simulink model "asenkronmodeli"  (Simulink 7.7)
settings: Solver=ode45  StartTime=0.0  StopTime=10.0  RelTol=1e-3
values from neighbouring files (symbols this model uses):
  J = 0.0226    [asenkronparametreler.m]
  p = 4    [asenkronparametreler.m]
  Rr = .39    (= 0.39)    [asenkronparametreler.m]
  Rs = .19    (= 0.19)    [asenkronparametreler.m]
  wb = 2*pi*fb    (= 628.318530718)    [asenkronparametreler.m]
  Xlr = wb*Llr    (= 0.376991118431)    [asenkronparametreler.m]
  Xls = wb*Lls    (= 0.131946891451)    [asenkronparametreler.m]
  Xmstar = 1/(1/Xls+1/Xm+1/Xlr)    (= 0.0940797800005)    [asenkronparametreler.m]
settings Model: Creator=Murat  LastModifiedBy=Murat
settings DataIOCC: SignalLoggingSaveFormat=Dataset
settings OptimizationCC: ExpressionDepthLimit=128
settings DebuggingCC: UnderspecifiedInitializationDetection=Simplified  MergeDetectMultiDrivingBlocksExec=error  FcnCallInpInsideContextMsg=Enable All  StateNameClashWarn=none
settings CodeAppCC: CustomSymbolStrType=$N$R$M_T
settings GRTTargetCC: TargetFunctionLibrary=C89/C90 (ANSI)

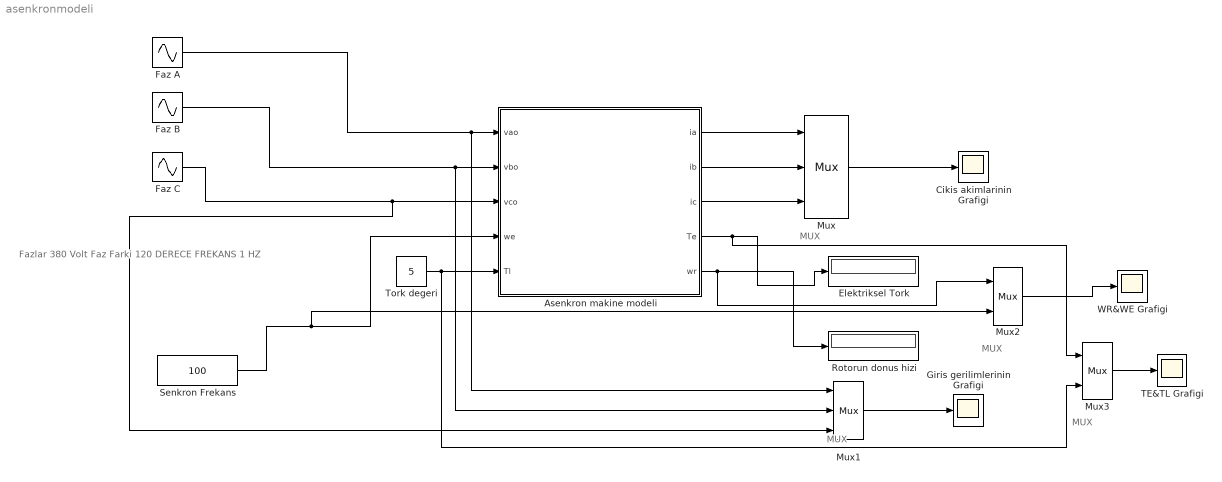
== system asenkronmodeli ==
  note: MUX
  note: MUX
  note: MUX
  note: MUX
  note: Fazlar 380 Volt
      | Faz Farki 120 DERECE
      | FREKANS 1 HZ
  Asenkron makine modeli : Subsystem
  Cikis akimlarinin Grafigi : Scope
      settings: SaveName=ScopeData3
  Elektriksel Tork : Display
  Faz A : Sin  Amplitude=380  SampleTime=0
  Faz B : Sin  Amplitude=380  Phase=(2*pi)/3  SampleTime=0
  Faz C : Sin  Amplitude=380  Phase=(4*pi)/3  SampleTime=0
  Giris gerilimlerinin Grafigi : Scope
      settings: SaveName=ScopeData4
  Mux : Mux  Inputs=3
  Mux1 : Mux  Inputs=3
  Mux2 : Mux  Inputs=2
  Mux3 : Mux  Inputs=2
  Rotorun donus hizi : Display
  Senkron Frekans : Constant  Value=100
  TE&TL Grafigi : Scope
      settings: SaveName=ScopeData5
  Tork degeri : Constant  Value=5
  WR&WE Grafigi : Scope
      settings: SaveName=ScopeData6
  wires:
  Asenkron makine modeli/1(ia) -> Mux/1
  Asenkron makine modeli/2(ib) -> Mux/2
  Asenkron makine modeli/3(ic) -> Mux/3
  Mux/1 -> Cikis akimlarinin Grafigi/1
  Asenkron makine modeli/5(wr) -> Mux2/1, Rotorun donus hizi/1
  Asenkron makine modeli/4(Te) -> Mux3/1, Elektriksel Tork/1
  Mux1/1 -> Giris gerilimlerinin Grafigi/1
  Tork degeri/1 -> Mux3/2, Asenkron makine modeli/5(Tl)
  Senkron Frekans/1 -> Mux2/2, Asenkron makine modeli/4(we)
  Faz A/1 -> Mux1/1, Asenkron makine modeli/1(vao)
  Faz B/1 -> Mux1/2, Asenkron makine modeli/2(vbo)
  Faz C/1 -> Mux1/3, Asenkron makine modeli/3(vco)
  Mux2/1 -> WR&WE Grafigi/1
  Mux3/1 -> TE&TL Grafigi/1

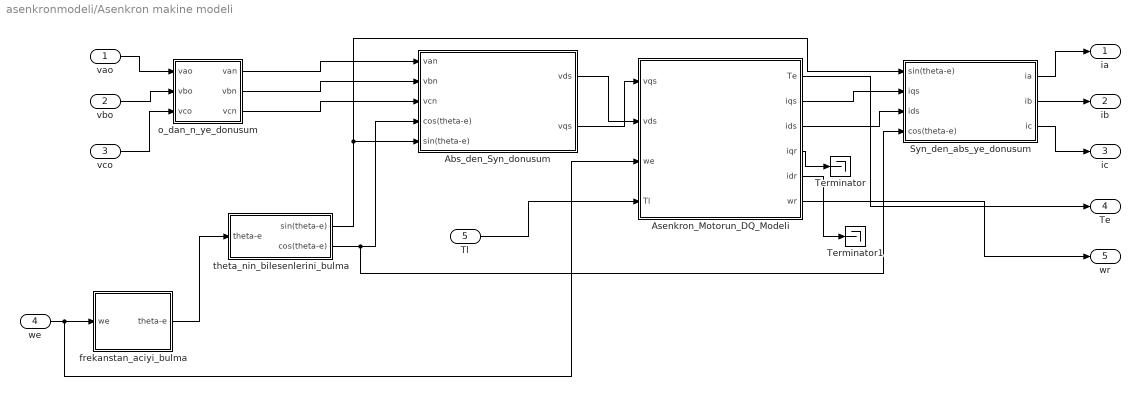
== system asenkronmodeli/Asenkron makine modeli ==
  vao : Inport
  vbo : Inport  Port=2
  vco : Inport  Port=3
  we : Inport  Port=4
  Tl : Inport  Port=5
  Abs_den_Syn_donusum : Subsystem
  Asenkron_Motorun_DQ_Modeli : Subsystem
  Syn_den_abs_ye_donusum : Subsystem
  Terminator : Terminator
  Terminator1 : Terminator
  frekanstan_aciyi_bulma : Subsystem
  o_dan_n_ye_donusum : Subsystem
  theta_nin_bilesenlerini_bulma : Subsystem
  ia : Outport
  ib : Outport  Port=2
  ic : Outport  Port=3
  Te : Outport  Port=4
  wr : Outport  Port=5
  wires:
  vbo/1 -> o_dan_n_ye_donusum/2(vbo)
  vao/1 -> o_dan_n_ye_donusum/1(vao)
  vco/1 -> o_dan_n_ye_donusum/3(vco)
  we/1 -> Asenkron_Motorun_DQ_Modeli/3(we), frekanstan_aciyi_bulma/1(we)
  frekanstan_aciyi_bulma/1(theta-e) -> theta_nin_bilesenlerini_bulma/1(theta-e)
  Asenkron_Motorun_DQ_Modeli/3(ids) -> Syn_den_abs_ye_donusum/3(ids)
  Syn_den_abs_ye_donusum/1(ia) -> ia/1
  Asenkron_Motorun_DQ_Modeli/4(iqr) -> Terminator/1
  Asenkron_Motorun_DQ_Modeli/5(idr) -> Terminator1/1
  Syn_den_abs_ye_donusum/3(ic) -> ic/1
  o_dan_n_ye_donusum/3(vcn) -> Abs_den_Syn_donusum/3(vcn)
  Asenkron_Motorun_DQ_Modeli/2(iqs) -> Syn_den_abs_ye_donusum/2(iqs)
  Abs_den_Syn_donusum/1(vds) -> Asenkron_Motorun_DQ_Modeli/2(vds)
  Abs_den_Syn_donusum/2(vqs) -> Asenkron_Motorun_DQ_Modeli/1(vqs)
  Syn_den_abs_ye_donusum/2(ib) -> ib/1
  Tl/1 -> Asenkron_Motorun_DQ_Modeli/4(Tl)
  o_dan_n_ye_donusum/2(vbn) -> Abs_den_Syn_donusum/2(vbn)
  o_dan_n_ye_donusum/1(van) -> Abs_den_Syn_donusum/1(van)
  Asenkron_Motorun_DQ_Modeli/1(Te) -> Te/1
  Asenkron_Motorun_DQ_Modeli/6(wr) -> wr/1
  theta_nin_bilesenlerini_bulma/2("cos(theta-e)   ") -> Syn_den_abs_ye_donusum/4("cos(theta-e) "), Abs_den_Syn_donusum/4("cos(theta-e) ")
  theta_nin_bilesenlerini_bulma/1("sin(theta-e)  ") -> Syn_den_abs_ye_donusum/1("sin(theta-e)  "), Abs_den_Syn_donusum/5(sin(theta-e))

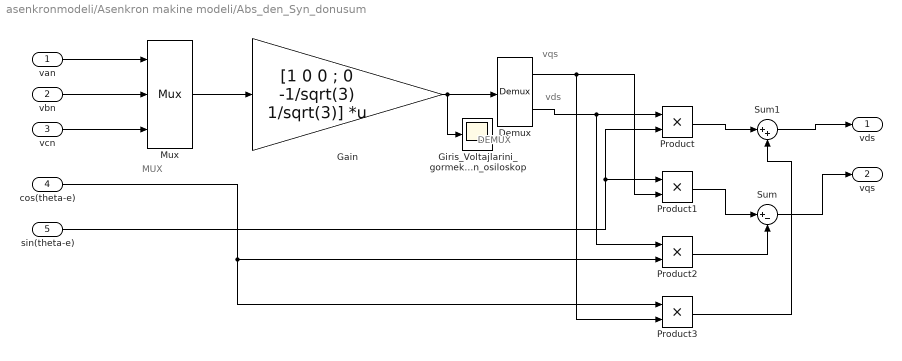
== system asenkronmodeli/Asenkron makine modeli/Abs_den_Syn_donusum ==
  note: vds
  note: vqs
  note: DEMUX
  note: MUX
  van : Inport
  vbn : Inport  Port=2
  vcn : Inport  Port=3
  "cos(theta-e) " : Inport  Port=4
  sin(theta-e) : Inport  Port=5
  Demux : Demux  Outputs=2
  Gain : Gain  Gain="[1 0 0 ; 0 -1/sqrt(3)  1/sqrt(3)]"  Multiplication=Matrix(K*u)  SaturateOnIntegerOverflow=on
  Giris_Voltajlarini_gormek_icin_osiloskop : Scope
  Mux : Mux  Inputs=3
  Product{,1..3} (4 alike) : Product
  Sum : Sum  Inputs=|+-
  Sum1 : Sum  Inputs=|++
  vds : Outport
  vqs : Outport  Port=2
  wires:
  van/1 -> Mux/1
  vbn/1 -> Mux/2
  vcn/1 -> Mux/3
  Mux/1 -> Gain/1
  Gain/1 -> Demux/1, Giris_Voltajlarini_gormek_icin_osiloskop/1
  sin(theta-e)/1 -> Product/2, Product1/1
  "cos(theta-e) "/1 -> Product3/1, Product2/2
  Demux/1 -> Product3/2, Product1/2
  Demux/2 -> Product2/1, Product/1
  Product2/1 -> Sum/2
  Product1/1 -> Sum/1
  Product/1 -> Sum1/1
  Product3/1 -> Sum1/2
  Sum1/1 -> vds/1
  Sum/1 -> vqs/1

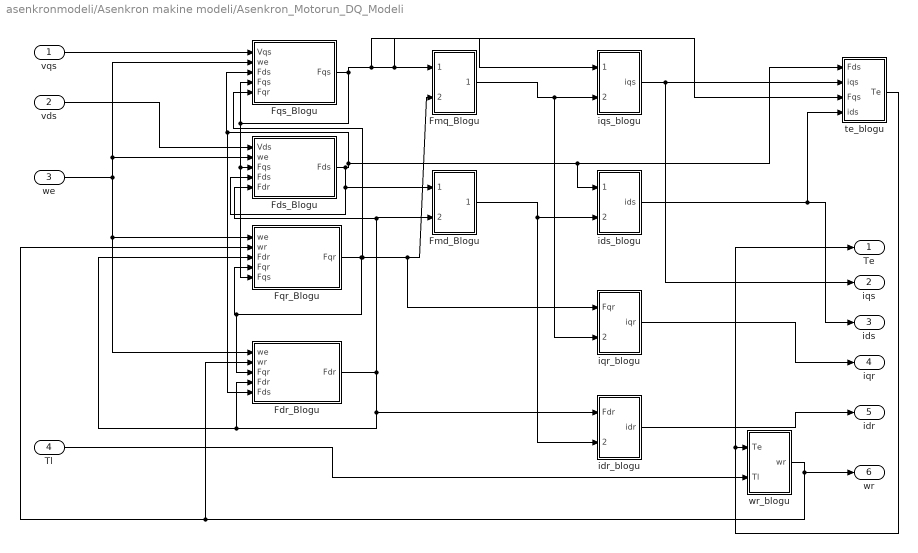
== system asenkronmodeli/Asenkron makine modeli/Asenkron_Motorun_DQ_Modeli ==
  vqs : Inport
  vds : Inport  Port=2
  we : Inport  Port=3
  Tl : Inport  Port=4
  Fdr_Blogu : Subsystem
  Fds_Blogu : Subsystem
  Fmd_Blogu : Subsystem
  Fmq_Blogu : Subsystem
  Fqr_Blogu : Subsystem
  Fqs_Blogu : Subsystem
  idr_blogu : Subsystem
  ids_blogu : Subsystem
  iqr_blogu : Subsystem
  iqs_blogu : Subsystem
  te_blogu : Subsystem
  wr_blogu : Subsystem
  Te : Outport
  iqs : Outport  Port=2
  ids : Outport  Port=3
  iqr : Outport  Port=4
  idr : Outport  Port=5
  wr : Outport  Port=6
  wires:
  vqs/1 -> Fqs_Blogu/1(Vqs)
  vds/1 -> Fds_Blogu/1("Vds ")
  we/1 -> Fds_Blogu/2(we), Fqs_Blogu/2(we), Fdr_Blogu/1("we "), Fqr_Blogu/1("we ")
  Tl/1 -> wr_blogu/2(Tl)
  Fqs_Blogu/1("Fqs   ") -> Fqr_Blogu/5(Fqs), Fds_Blogu/3("Fqs  "), Fqs_Blogu/4(Fqs), te_blogu/3("Fqs  "), iqs_blogu/1(Fqs), Fmq_Blogu/1("Fqs  ")
  Fds_Blogu/1("Fds   ") -> Fmd_Blogu/1("Fds  "), Fds_Blogu/4(Fds), te_blogu/1("Fds   "), ids_blogu/1("Fds  "), Fdr_Blogu/5(Fds), Fqs_Blogu/3(Fds)
  Fqr_Blogu/1("Fqr  ") -> iqr_blogu/1("Fqr  "), Fmq_Blogu/2("Fqr  "), Fqs_Blogu/5(Fqr), Fdr_Blogu/3("Fqr   "), Fqr_Blogu/4(Fqr)
  Fdr_Blogu/1("Fdr  ") -> idr_blogu/1("Fdr  "), Fqr_Blogu/3("Fdr  "), Fdr_Blogu/4(Fdr), Fmd_Blogu/2("Fdr  "), Fds_Blogu/5(Fdr)
  wr_blogu/1(wr) -> wr/1, Fdr_Blogu/2(wr), Fqr_Blogu/2(wr)
  Fmq_Blogu/1(Fmq) -> iqr_blogu/2("Fmq "), iqs_blogu/2(Fmq)
  Fmd_Blogu/1(Fmd) -> idr_blogu/2("Fmd "), ids_blogu/2("Fmd ")
  iqs_blogu/1(iqs) -> iqs/1, te_blogu/2(iqs)
  ids_blogu/1(ids) -> ids/1, te_blogu/4("ids ")
  te_blogu/1(Te) -> Te/1, wr_blogu/1(Te)
  idr_blogu/1(idr) -> idr/1
  iqr_blogu/1(iqr) -> iqr/1

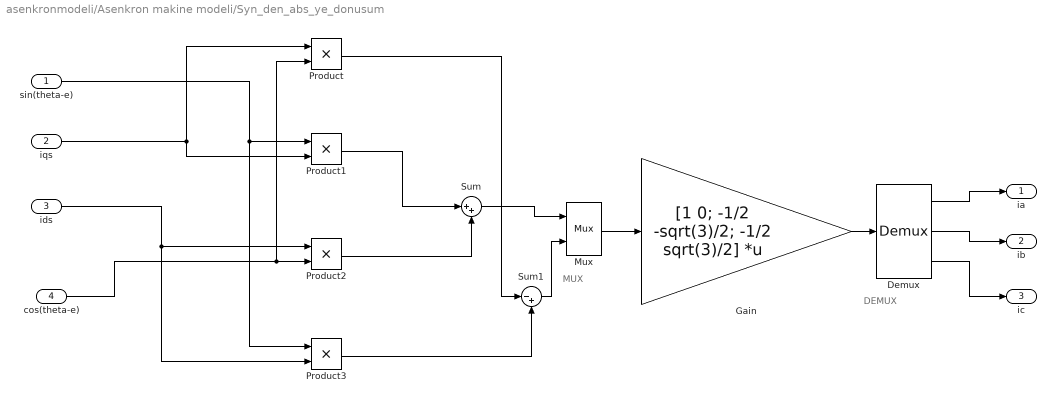
== system asenkronmodeli/Asenkron makine modeli/Syn_den_abs_ye_donusum ==
  note: DEMUX
  note: MUX
  "sin(theta-e)  " : Inport
  iqs : Inport  Port=2
  ids : Inport  Port=3
  "cos(theta-e) " : Inport  Port=4
  Demux : Demux  Outputs=3
  Gain : Gain  Gain="[1 0; -1/2 -sqrt(3)/2;  -1/2 sqrt(3)/2]"  Multiplication=Matrix(K*u)  SaturateOnIntegerOverflow=on
  Mux : Mux  Inputs=2
  Product{,1..3} (4 alike) : Product
  Sum : Sum  Inputs=|++
  Sum1 : Sum  Inputs=|-+
  ia : Outport
  ib : Outport  Port=2
  ic : Outport  Port=3
  wires:
  iqs/1 -> Product1/2, Product/1
  "sin(theta-e)  "/1 -> Product3/1, Product1/1
  ids/1 -> Product2/1, Product3/2
  "cos(theta-e) "/1 -> Product/2, Product2/2
  Product2/1 -> Sum/2
  Product1/1 -> Sum/1
  Product3/1 -> Sum1/2
  Product/1 -> Sum1/1
  Sum1/1 -> Mux/2
  Sum/1 -> Mux/1
  Mux/1 -> Gain/1
  Gain/1 -> Demux/1
  Demux/1 -> ia/1
  Demux/2 -> ib/1
  Demux/3 -> ic/1

== system asenkronmodeli/Asenkron makine modeli/frekanstan_aciyi_bulma ==
  we : Inport
  Constant : Constant  Value=2*pi
  Integrator : Integrator
  Math Function : Math  Operator=mod  SaturateOnIntegerOverflow=on
  theta-e : Outport
  wires:
  we/1 -> Integrator/1
  Integrator/1 -> Math Function/1
  Constant/1 -> Math Function/2
  Math Function/1 -> theta-e/1

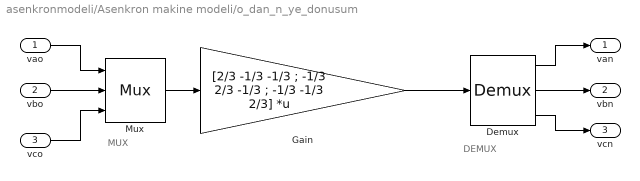
== system asenkronmodeli/Asenkron makine modeli/o_dan_n_ye_donusum ==
  note: DEMUX
  note: MUX
  vao : Inport
  vbo : Inport  Port=2
  vco : Inport  Port=3
  Demux : Demux  Outputs=3
  Gain : Gain  Gain=[2/3 -1/3 -1/3 ; -1/3 2/3 -1/3 ; -1/3 -1/3 2/3]  Multiplication=Matrix(K*u)
  Mux : Mux  Inputs=3
  van : Outport
  vbn : Outport  Port=2
  vcn : Outport  Port=3
  wires:
  Demux/3 -> vcn/1
  Gain/1 -> Demux/1
  vao/1 -> Mux/1
  Demux/1 -> van/1
  Mux/1 -> Gain/1
  Demux/2 -> vbn/1
  vco/1 -> Mux/3
  vbo/1 -> Mux/2

== system asenkronmodeli/Asenkron makine modeli/theta_nin_bilesenlerini_bulma ==
  theta-e : Inport
  Trigonometric Function : Trigonometry
  Trigonometric Function1 : Trigonometry  Operator=cos
  "sin(theta-e)  " : Outport
  "cos(theta-e)   " : Outport  Port=2
  wires:
  theta-e/1 -> Trigonometric Function1/1, Trigonometric Function/1
  Trigonometric Function1/1 -> "cos(theta-e)   "/1
  Trigonometric Function/1 -> "sin(theta-e)  "/1

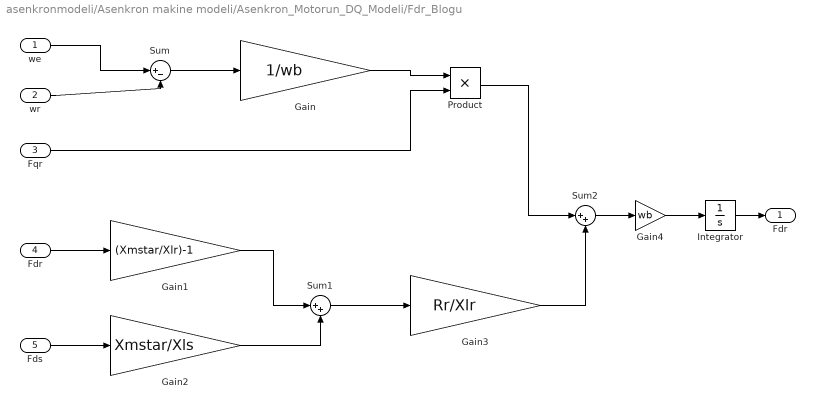
== system asenkronmodeli/Asenkron makine modeli/Asenkron_Motorun_DQ_Modeli/Fdr_Blogu ==
  "we " : Inport
  wr : Inport  Port=2
  "Fqr   " : Inport  Port=3
  Fdr : Inport  Port=4
  Fds : Inport  Port=5
  Gain : Gain  Gain=1/wb
  Gain1 : Gain  Gain=(Xmstar/Xlr)-1
  Gain2 : Gain  Gain=Xmstar/Xls
  Gain3 : Gain  Gain=Rr/Xlr
  Gain4 : Gain  Gain=wb  SaturateOnIntegerOverflow=on
  Integrator : Integrator
  Product : Product
  Sum : Sum  Inputs=|+-
  Sum1 : Sum  Inputs=|++
  Sum2 : Sum  Inputs=|++
  "Fdr  " : Outport
  wires:
  Sum/1 -> Gain/1
  wr/1 -> Sum/2
  "we "/1 -> Sum/1
  Gain/1 -> Product/1
  "Fqr   "/1 -> Product/2
  Gain1/1 -> Sum1/1
  Gain2/1 -> Sum1/2
  Fds/1 -> Gain2/1
  Fdr/1 -> Gain1/1
  Sum1/1 -> Gain3/1
  Product/1 -> Sum2/1
  Gain3/1 -> Sum2/2
  Sum2/1 -> Gain4/1
  Gain4/1 -> Integrator/1
  Integrator/1 -> "Fdr  "/1

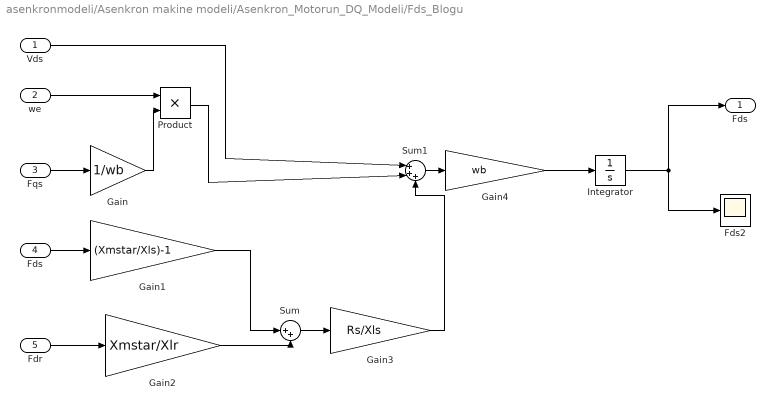
== system asenkronmodeli/Asenkron makine modeli/Asenkron_Motorun_DQ_Modeli/Fds_Blogu ==
  "Vds " : Inport
  we : Inport  Port=2
  "Fqs  " : Inport  Port=3
  Fds : Inport  Port=4
  Fdr : Inport  Port=5
  "Fds2   " : Scope
      settings: SaveName=ScopeData2
  Gain : Gain  Gain=1/wb
  Gain1 : Gain  Gain=(Xmstar/Xls)-1  SaturateOnIntegerOverflow=on
  Gain2 : Gain  Gain=Xmstar/Xlr
  Gain3 : Gain  Gain=Rs/Xls
  Gain4 : Gain  Gain=wb
  Integrator : Integrator
  Product : Product
  Sum : Sum  Inputs=|++
  Sum1 : Sum  Inputs=|+++
  "Fds   " : Outport
  wires:
  Integrator/1 -> "Fds   "/1, "Fds2   "/1
  Gain4/1 -> Integrator/1
  Gain3/1 -> Sum1/3
  Gain/1 -> Product/2
  Fds/1 -> Gain1/1
  Gain1/1 -> Sum/1
  "Vds "/1 -> Sum1/1
  we/1 -> Product/1
  Gain2/1 -> Sum/2
  Sum1/1 -> Gain4/1
  "Fqs  "/1 -> Gain/1
  Fdr/1 -> Gain2/1
  Sum/1 -> Gain3/1
  Product/1 -> Sum1/2

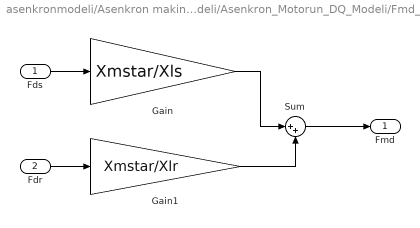
== system asenkronmodeli/Asenkron makine modeli/Asenkron_Motorun_DQ_Modeli/Fmd_Blogu ==
  "Fds  " : Inport
  "Fdr  " : Inport  Port=2
  Gain : Gain  Gain=Xmstar/Xls  SaturateOnIntegerOverflow=on
  Gain1 : Gain  Gain=Xmstar/Xlr
  Sum : Sum  Inputs=|++
  Fmd : Outport
  wires:
  "Fdr  "/1 -> Gain1/1
  "Fds  "/1 -> Gain/1
  Gain/1 -> Sum/1
  Sum/1 -> Fmd/1
  Gain1/1 -> Sum/2

== system asenkronmodeli/Asenkron makine modeli/Asenkron_Motorun_DQ_Modeli/Fmq_Blogu ==
  "Fqs  " : Inport
  "Fqr  " : Inport  Port=2
  Gain : Gain  Gain=Xmstar/Xls  SaturateOnIntegerOverflow=on
  Gain1 : Gain  Gain=Xmstar/Xlr
  Sum : Sum  Inputs=|++
  Fmq : Outport
  wires:
  "Fqs  "/1 -> Gain/1
  Gain/1 -> Sum/1
  Gain1/1 -> Sum/2
  "Fqr  "/1 -> Gain1/1
  Sum/1 -> Fmq/1

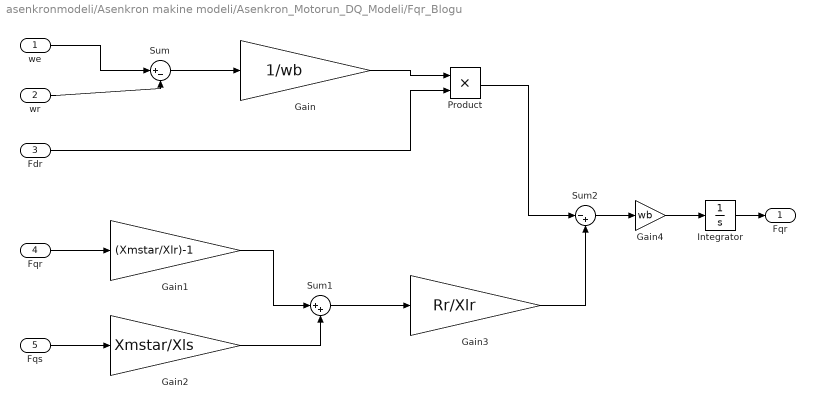
== system asenkronmodeli/Asenkron makine modeli/Asenkron_Motorun_DQ_Modeli/Fqr_Blogu ==
  "we " : Inport
  wr : Inport  Port=2
  "Fdr  " : Inport  Port=3
  Fqr : Inport  Port=4
  Fqs : Inport  Port=5
  Gain : Gain  Gain=1/wb
  Gain1 : Gain  Gain=(Xmstar/Xlr)-1
  Gain2 : Gain  Gain=Xmstar/Xls
  Gain3 : Gain  Gain=Rr/Xlr
  Gain4 : Gain  Gain=wb  SaturateOnIntegerOverflow=on
  Integrator : Integrator
  Product : Product
  Sum : Sum  Inputs=|+-
  Sum1 : Sum  Inputs=|++
  Sum2 : Sum  Inputs=|-+
  "Fqr  " : Outport
  wires:
  Sum/1 -> Gain/1
  wr/1 -> Sum/2
  "we "/1 -> Sum/1
  Gain/1 -> Product/1
  "Fdr  "/1 -> Product/2
  Gain1/1 -> Sum1/1
  Gain2/1 -> Sum1/2
  Fqs/1 -> Gain2/1
  Fqr/1 -> Gain1/1
  Sum1/1 -> Gain3/1
  Product/1 -> Sum2/1
  Gain3/1 -> Sum2/2
  Sum2/1 -> Gain4/1
  Gain4/1 -> Integrator/1
  Integrator/1 -> "Fqr  "/1

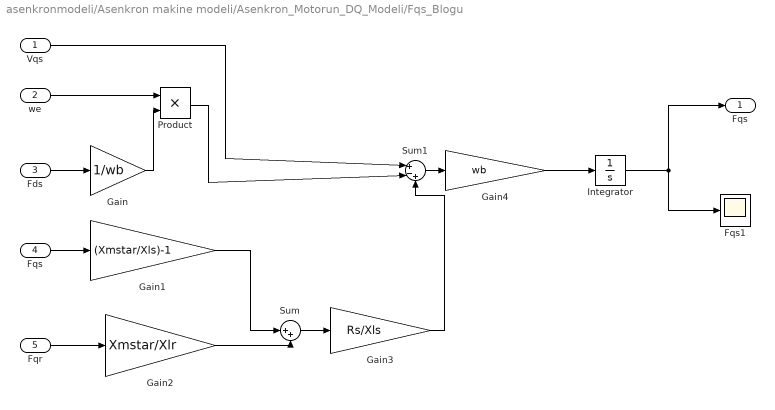
== system asenkronmodeli/Asenkron makine modeli/Asenkron_Motorun_DQ_Modeli/Fqs_Blogu ==
  Vqs : Inport
  we : Inport  Port=2
  Fds : Inport  Port=3
  Fqs : Inport  Port=4
  Fqr : Inport  Port=5
  "Fqs1   " : Scope
  Gain : Gain  Gain=1/wb
  Gain1 : Gain  Gain=(Xmstar/Xls)-1  SaturateOnIntegerOverflow=on
  Gain2 : Gain  Gain=Xmstar/Xlr
  Gain3 : Gain  Gain=Rs/Xls
  Gain4 : Gain  Gain=wb
  Integrator : Integrator
  Product : Product
  Sum : Sum  Inputs=|++
  Sum1 : Sum  Inputs=|+-+
  "Fqs   " : Outport
  wires:
  Integrator/1 -> "Fqs   "/1, "Fqs1   "/1
  Gain4/1 -> Integrator/1
  Gain3/1 -> Sum1/3
  Gain/1 -> Product/2
  Fqs/1 -> Gain1/1
  Gain1/1 -> Sum/1
  Vqs/1 -> Sum1/1
  we/1 -> Product/1
  Gain2/1 -> Sum/2
  Sum1/1 -> Gain4/1
  Fds/1 -> Gain/1
  Fqr/1 -> Gain2/1
  Sum/1 -> Gain3/1
  Product/1 -> Sum1/2

== system asenkronmodeli/Asenkron makine modeli/Asenkron_Motorun_DQ_Modeli/idr_blogu ==
  "Fdr  " : Inport
  "Fmd " : Inport  Port=2
  Gain : Gain  Gain=1/Xlr
  Sum : Sum  Inputs=|+-
  idr : Outport
  wires:
  "Fdr  "/1 -> Sum/1
  Gain/1 -> idr/1
  Sum/1 -> Gain/1
  "Fmd "/1 -> Sum/2

== system asenkronmodeli/Asenkron makine modeli/Asenkron_Motorun_DQ_Modeli/ids_blogu ==
  "Fds  " : Inport
  "Fmd " : Inport  Port=2
  Gain : Gain  Gain=1/Xls
  Sum : Sum  Inputs=|+-
  ids : Outport
  wires:
  "Fds  "/1 -> Sum/1
  Gain/1 -> ids/1
  "Fmd "/1 -> Sum/2
  Sum/1 -> Gain/1

== system asenkronmodeli/Asenkron makine modeli/Asenkron_Motorun_DQ_Modeli/iqr_blogu ==
  "Fqr  " : Inport
  "Fmq " : Inport  Port=2
  Gain : Gain  Gain=1/Xlr
  Sum : Sum  Inputs=|+-
  iqr : Outport
  wires:
  "Fqr  "/1 -> Sum/1
  Gain/1 -> iqr/1
  Sum/1 -> Gain/1
  "Fmq "/1 -> Sum/2

== system asenkronmodeli/Asenkron makine modeli/Asenkron_Motorun_DQ_Modeli/iqs_blogu ==
  Fqs : Inport
  Fmq : Inport  Port=2
  Gain : Gain  Gain=1/Xls
  Sum : Sum  Inputs=|+-
  iqs : Outport
  wires:
  Gain/1 -> iqs/1
  Fqs/1 -> Sum/1
  Fmq/1 -> Sum/2
  Sum/1 -> Gain/1

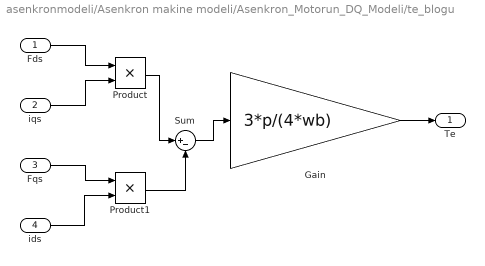
== system asenkronmodeli/Asenkron makine modeli/Asenkron_Motorun_DQ_Modeli/te_blogu ==
  "Fds   " : Inport
  iqs : Inport  Port=2
  "Fqs  " : Inport  Port=3
  "ids " : Inport  Port=4
  Gain : Gain  Gain=3*p/(4*wb)
  Product : Product
  Product1 : Product
  Sum : Sum  Inputs=|+-
  Te : Outport
  wires:
  "ids "/1 -> Product1/2
  Sum/1 -> Gain/1
  "Fqs  "/1 -> Product1/1
  Product/1 -> Sum/1
  Gain/1 -> Te/1
  Product1/1 -> Sum/2
  "Fds   "/1 -> Product/1
  iqs/1 -> Product/2

== system asenkronmodeli/Asenkron makine modeli/Asenkron_Motorun_DQ_Modeli/wr_blogu ==
  Te : Inport
  Tl : Inport  Port=2
  Gain : Gain  Gain=p/(2*J)
  Integrator : Integrator
  Sum : Sum  Inputs=|+-
  wr : Outport
  wires:
  Te/1 -> Sum/1
  Sum/1 -> Gain/1
  Tl/1 -> Sum/2
  Integrator/1 -> wr/1
  Gain/1 -> Integrator/1
